simulink model "REGACCESSDEMO"  (R2014b)
settings: Solver=FixedStepDiscrete  StartTime=0.0  StopTime=10.0  FixedStep=1e-3  RelTol=1e-3
PreLoadFcn:
  | Hyo_customization
libraries: periblklib x4
settings Model: Creator=sunzx.fnst  LastModifiedBy=sunzx.fnst
settings DataIOCC: SaveFormat=Structure
settings OptimizationCC: InlineParams=on  OptimizeModelRefInitCode=on  LifeSpan=1
settings HardwareCC: ProdLargestAtomicInteger=Integer  ProdLargestAtomicFloat=Float  ProdIntDivRoundTo=Zero  ProdEndianess=LittleEndian  ProdHWDeviceType=CYPRESS->ARM Cortex-R5
settings RTWCC: SystemTargetFile=Hyo.tlc  GenCodeOnly=on  MakeCommand=none  GenerateMakefile=off  TemplateMakefile=none  Description=System Target File for S6J3200 Series MCU Target  GenerateReport=on  ProcessScript=Hyo_make_rtw_hook  IncludeHyperlinkInReport=on  LaunchReport=on
settings CodeAppCC: IgnoreCustomStorageClasses=off
settings STFCustomTargetCC: ModelReferenceCompliant=off  IncludeMdlTerminateFcn=off  CombineOutputUpdateFcns=on  ERTFirstTimeCompliant=on  ERTCustomFileBanners=on  SupportContinuousTime=off  SupportNonInlinedSFcns=off  MATLABClassNameForMDSCustomization=Simulink.SoftwareTarget.ERTCustomization  GRTInterface=off  SystemTargetFile=Hyo.tlc
settings ERTTargetCC: ModelReferenceCompliant=off  ParMdlRefBuildCompliant=off  CompOptLevelCompliant=off  ConcurrentExecutionCompliant=off  IncludeMdlTerminateFcn=off  ModelStepFunctionPrototypeControlCompliant=off  CPPClassGenCompliant=off  InlinedParameterPlacement=NonHierarchical  ERTSrcFileBannerTemplate=Hyo_code_template.cgt  ERTHdrFileBannerTemplate=Hyo_code_template.cgt  ERTDataSrcFileTemplate=Hyo_code_template.cgt  ERTDataHdrFileTemplate=Hyo_code_template.cgt  ERTCustomFileTemplate=example_file_process.tlc  EnableUserReplacementTypes=on

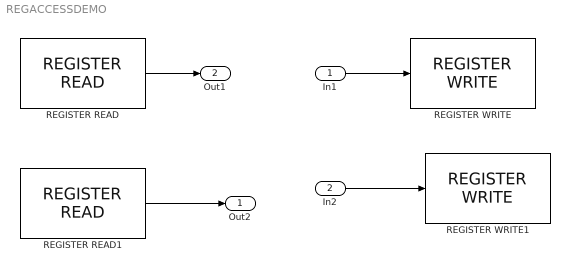
== system REGACCESSDEMO ==
  In1 : Inport
  In2 : Inport  Port=2
  REGISTER READ : periblklib/Register Access/REGISTER READ  g_pv=s6j3200io.h,REGISTER,_Read_QC08_QICRL_ZIIF;peri,QC;reg,QC08_QICRL_ZIIF;invisiblecontrol,unsigned char ;
  REGISTER READ1 : periblklib/Register Access/REGISTER READ  g_pv=s6j3200io.h,REGISTER,_Read_SADAC_DAOSR_OSR;peri,SADAC;reg,SADAC_DAOSR_OSR;invisiblecontrol,uint_io8_t ;
  REGISTER WRITE : periblklib/Register Access/REGISTER WRITE  g_pv=s6j3200io.h,REGISTER,_Write_SWDG_RSTCAUSE_RSTCAUSE0;peri,SWDG;reg,SWDG_RSTCAUSE_RSTCAUSE0;invisiblecontrol,uint_io16_t ;
  REGISTER WRITE1 : periblklib/Register Access/REGISTER WRITE  g_pv=s6j3200io.h,REGISTER,_Write_ADC12B0_CHCTRL2_RSMRST;peri,ADC12B;reg,ADC12B0_CHCTRL2_RSMRST;invisiblecontrol,uint_io8_t ;
  Out2 : Outport
  Out1 : Outport  Port=2
  wires:
  REGISTER READ1/1 -> Out2/1
  REGISTER READ/1 -> Out1/1
  In1/1 -> REGISTER WRITE/1
  In2/1 -> REGISTER WRITE1/1
